simulink model "HybridFilter"  (R2022b)
settings: Solver=FixedStepDiscrete  StartTime=0.0  StopTime=10.0  RelTol=1e-3
libraries: simulink x1
settings Model: Creator=yuzehong  LastModifiedBy=yuzehong
settings OptimizationCC: DefaultParameterBehavior=Inlined  UseDivisionForNetSlopeComputation=on  GainParamInheritBuiltInType=on  UseFloatMulNetSlope=on  InlineInvariantSignals=on  PassReuseOutputArgsAs=Individual arguments  NoFixptDivByZeroProtection=on  EfficientFloat2IntCast=on  LifeSpan=1  OptimizeBlockOrder=speed  DifferentSizesBufferReuse=on  EfficientTunableParamExpr=on
settings DebuggingCC: ParameterTunabilityLossMsg=error
settings HardwareCC: ProdLongLongMode=on
settings SFSimCC: MATLABDynamicMemAlloc=off
settings RTWCC: Description=Embedded Coder  SystemTargetFile=ert.tlc  TemplateMakefile=ert_default_tmf
settings CodeAppCC: GenerateComments=off  IgnoreCustomStorageClasses=off  OperatorAnnotations=on  SimulinkDataObjDesc=on  SFDataObjDesc=on  CustomSymbolStrGlobalVar=rt$N$M  CustomSymbolStrType=$N$M  CustomSymbolStrFcn=$N$M$F  CustomSymbolStrMacro=$N$M  SimulinkBlockComments=off
settings ERTTargetCC: TargetLangStandard=C99 (ISO)  GenerateSampleERTMain=on  IncludeMdlTerminateFcn=off  CombineSignalStateStructs=on  SupportAbsoluteTime=off  CodeInterfacePackaging=Reusable function  SupportComplex=off  SupportNonInlinedSFcns=on  InlinedParameterPlacement=NonHierarchical  ERTCustomFileTemplate=example_file_process.tlc  ERTFilePackagingFormat=CompactWithDataFile

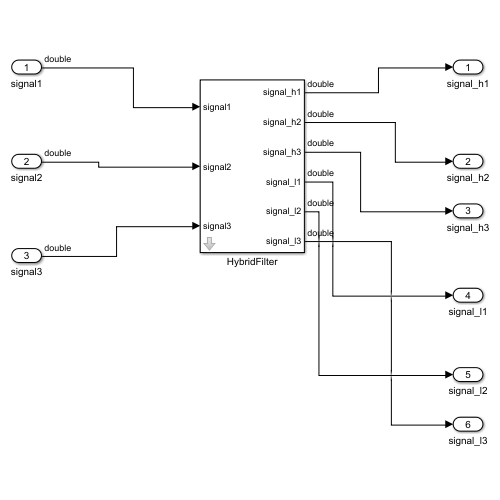
[thumbnail: Simulink's stored preview of the top-level diagram]
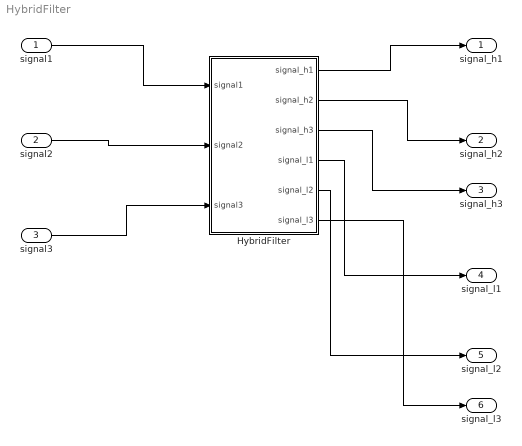
== system HybridFilter ==
  signal1 : Inport  OutDataTypeStr=double  PortDimensions=32
  signal2 : Inport  Port=2  OutDataTypeStr=double  PortDimensions=32
  signal3 : Inport  Port=3  OutDataTypeStr=double  PortDimensions=32
  HybridFilter : Subsystem  mask{length=32}
      mask DialogControl ParameterGroupVar Prompt: 参数
  signal_h1 : Outport
  signal_h2 : Outport  Port=2
  signal_h3 : Outport  Port=3
  signal_l1 : Outport  Port=4
  signal_l2 : Outport  Port=5
  signal_l3 : Outport  Port=6
  wires:
  signal1/1 -> HybridFilter/1(signal1)
  signal2/1 -> HybridFilter/2(signal2)
  signal3/1 -> HybridFilter/3(signal3)
  HybridFilter/1(signal_h1) -> signal_h1/1
  HybridFilter/2(signal_h2) -> signal_h2/1
  HybridFilter/3(signal_h3) -> signal_h3/1
  HybridFilter/4(signal_l1) -> signal_l1/1
  HybridFilter/5(signal_l2) -> signal_l2/1
  HybridFilter/6(signal_l3) -> signal_l3/1

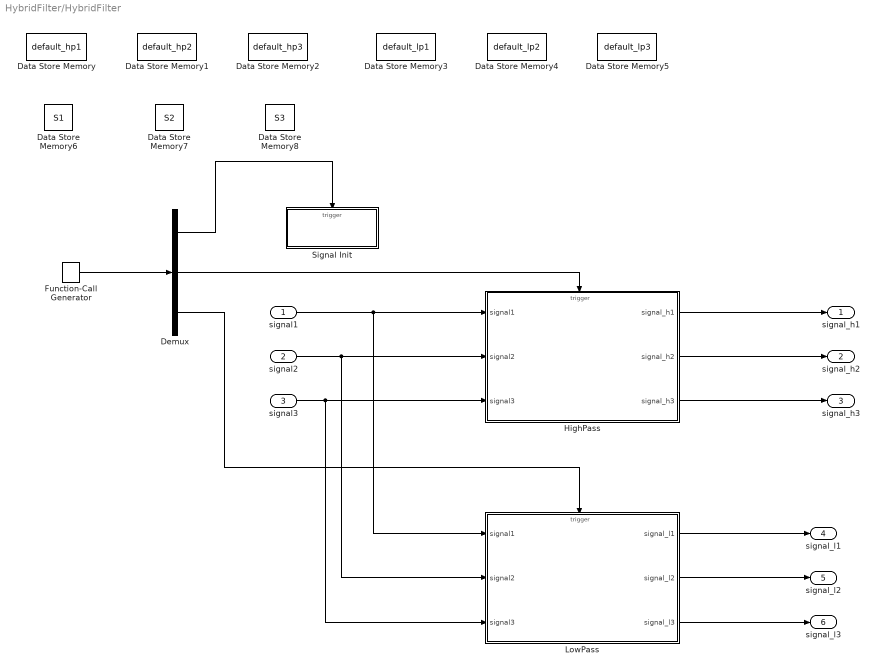
== system HybridFilter/HybridFilter ==
  signal1 : Inport  PortDimensions=length
  signal2 : Inport  Port=2  PortDimensions=length
  signal3 : Inport  Port=3  PortDimensions=length
  Data Store Memory : DataStoreMemory  DataStoreName=default_hp1  WriteAfterWriteMsg=warning  ShowAdditionalParam=off
  Data Store Memory1 : DataStoreMemory  DataStoreName=default_hp2  WriteAfterWriteMsg=warning  ShowAdditionalParam=off
  Data Store Memory2 : DataStoreMemory  DataStoreName=default_hp3  WriteAfterWriteMsg=warning  ShowAdditionalParam=off
  Data Store Memory3 : DataStoreMemory  DataStoreName=default_lp1  WriteAfterWriteMsg=warning  ShowAdditionalParam=off
  Data Store Memory4 : DataStoreMemory  DataStoreName=default_lp2  WriteAfterWriteMsg=warning  ShowAdditionalParam=off
  Data Store Memory5 : DataStoreMemory  DataStoreName=default_lp3  WriteAfterWriteMsg=warning  ShowAdditionalParam=off
  Data Store Memory6 : DataStoreMemory  DataStoreName=S1  WriteAfterWriteMsg=warning  ShowAdditionalParam=off  OutDataTypeStr=double  Dimensions=length
  Data Store Memory7 : DataStoreMemory  DataStoreName=S2  WriteAfterWriteMsg=warning  ShowAdditionalParam=off  OutDataTypeStr=double  Dimensions=length
  Data Store Memory8 : DataStoreMemory  DataStoreName=S3  WriteAfterWriteMsg=warning  ShowAdditionalParam=off  OutDataTypeStr=double  Dimensions=length
  Demux : Demux  Outputs=3
  Function-Call Generator : simulink/Ports & Subsystems/Function-Call Generator  sample_time=1  numberOfIterations=1  DisallowWideOutput=off
  HighPass : Subsystem
  LowPass : Subsystem
  Signal Init : Subsystem  TreatAsAtomicUnit=on
  signal_h1 : Outport
  signal_h2 : Outport  Port=2
  signal_h3 : Outport  Port=3
  signal_l1 : Outport  Port=4
  signal_l2 : Outport  Port=5
  signal_l3 : Outport  Port=6
  wires:
  Function-Call Generator/1 -> Demux/1
  Demux/1 -> Signal Init/Trigger
  signal1/1 -> LowPass/1(signal1), HighPass/1(signal1)
  signal2/1 -> LowPass/2(signal2), HighPass/2(signal2)
  signal3/1 -> LowPass/3(signal3), HighPass/3(signal3)
  HighPass/1(signal_h1) -> signal_h1/1
  HighPass/2(signal_h2) -> signal_h2/1
  HighPass/3(signal_h3) -> signal_h3/1
  Demux/2 -> HighPass/Trigger
  Demux/3 -> LowPass/Trigger
  LowPass/1(signal_l1) -> signal_l1/1
  LowPass/2(signal_l2) -> signal_l2/1
  LowPass/3(signal_l3) -> signal_l3/1

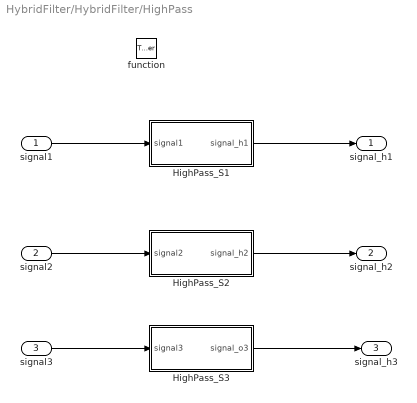
== system HybridFilter/HybridFilter/HighPass ==
  signal1 : Inport
  signal2 : Inport  Port=2
  signal3 : Inport  Port=3
  function : TriggerPort  TriggerType=function-call  VariantControl=(inherit)
  HighPass_S1 : Subsystem  TreatAsAtomicUnit=on
  HighPass_S2 : Subsystem  TreatAsAtomicUnit=on
  HighPass_S3 : Subsystem  TreatAsAtomicUnit=on
  signal_h1 : Outport
  signal_h2 : Outport  Port=2
  signal_h3 : Outport  Port=3
  wires:
  HighPass_S1/1(signal_h1) -> signal_h1/1
  HighPass_S2/1(signal_h2) -> signal_h2/1
  HighPass_S3/1(signal_o3) -> signal_h3/1
  signal1/1 -> HighPass_S1/1(signal1)
  signal2/1 -> HighPass_S2/1(signal2)
  signal3/1 -> HighPass_S3/1(signal3)

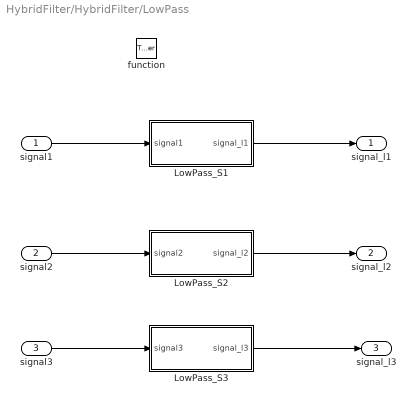
== system HybridFilter/HybridFilter/LowPass ==
  signal1 : Inport
  signal2 : Inport  Port=2
  signal3 : Inport  Port=3
  function : TriggerPort  TriggerType=function-call  VariantControl=(inherit)
  LowPass_S1 : Subsystem  TreatAsAtomicUnit=on
  LowPass_S2 : Subsystem  TreatAsAtomicUnit=on
  LowPass_S3 : Subsystem  TreatAsAtomicUnit=on
  signal_l1 : Outport
  signal_l2 : Outport  Port=2
  signal_l3 : Outport  Port=3
  wires:
  LowPass_S1/1(signal_l1) -> signal_l1/1
  LowPass_S2/1(signal_l2) -> signal_l2/1
  LowPass_S3/1(signal_l3) -> signal_l3/1
  signal1/1 -> LowPass_S1/1(signal1)
  signal2/1 -> LowPass_S2/1(signal2)
  signal3/1 -> LowPass_S3/1(signal3)

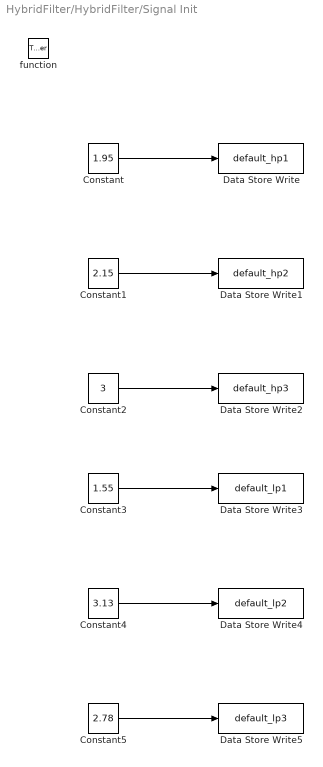
== system HybridFilter/HybridFilter/Signal Init ==
  function : TriggerPort  TriggerType=function-call  VariantControl=(inherit)
  Constant : Constant  Value=1.95  OutDataTypeStr=single
  Constant1 : Constant  Value=2.15  OutDataTypeStr=single
  Constant2 : Constant  Value=3  OutDataTypeStr=single
  Constant3 : Constant  Value=1.55  OutDataTypeStr=single
  Constant4 : Constant  Value=3.13  OutDataTypeStr=single
  Constant5 : Constant  Value=2.78  OutDataTypeStr=single
  Data Store Write : DataStoreWrite  DataStoreName=default_hp1  IndexOptions=Index vector (dialog)  Indices=1  OutputSizes=1
  Data Store Write1 : DataStoreWrite  DataStoreName=default_hp2  IndexOptions=Index vector (dialog)  Indices=1  OutputSizes=1
  Data Store Write2 : DataStoreWrite  DataStoreName=default_hp3  IndexOptions=Index vector (dialog)  Indices=1  OutputSizes=1
  Data Store Write3 : DataStoreWrite  DataStoreName=default_lp1  IndexOptions=Index vector (dialog)  Indices=1  OutputSizes=1
  Data Store Write4 : DataStoreWrite  DataStoreName=default_lp2  IndexOptions=Index vector (dialog)  Indices=1  OutputSizes=1
  Data Store Write5 : DataStoreWrite  DataStoreName=default_lp3  IndexOptions=Index vector (dialog)  Indices=1  OutputSizes=1
  wires:
  Constant/1 -> Data Store Write/1
  Constant1/1 -> Data Store Write1/1
  Constant2/1 -> Data Store Write2/1
  Constant5/1 -> Data Store Write5/1
  Constant4/1 -> Data Store Write4/1
  Constant3/1 -> Data Store Write3/1

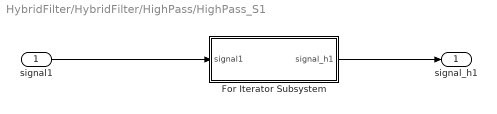
== system HybridFilter/HybridFilter/HighPass/HighPass_S1 ==
  signal1 : Inport
  For Iterator Subsystem : Subsystem  TreatAsAtomicUnit=on
  signal_h1 : Outport
  wires:
  signal1/1 -> For Iterator Subsystem/1(signal1)
  For Iterator Subsystem/1(signal_h1) -> signal_h1/1

== system HybridFilter/HybridFilter/HighPass/HighPass_S2 ==
  signal2 : Inport
  For Iterator Subsystem : Subsystem  TreatAsAtomicUnit=on
  signal_h2 : Outport
  wires:
  signal2/1 -> For Iterator Subsystem/1(signal2)
  For Iterator Subsystem/1(signal_h2) -> signal_h2/1

== system HybridFilter/HybridFilter/HighPass/HighPass_S3 ==
  signal3 : Inport
  For Iterator Subsystem : Subsystem  TreatAsAtomicUnit=on
  signal_o3 : Outport
  wires:
  For Iterator Subsystem/1(signal_o3) -> signal_o3/1
  signal3/1 -> For Iterator Subsystem/1(signal3)

== system HybridFilter/HybridFilter/LowPass/LowPass_S1 ==
  signal1 : Inport
  For Iterator Subsystem : Subsystem  TreatAsAtomicUnit=on
  signal_l1 : Outport
  wires:
  signal1/1 -> For Iterator Subsystem/1(signal1)
  For Iterator Subsystem/1(signal_l1) -> signal_l1/1

== system HybridFilter/HybridFilter/LowPass/LowPass_S2 ==
  signal2 : Inport
  For Iterator Subsystem : Subsystem  TreatAsAtomicUnit=on
  signal_l2 : Outport
  wires:
  signal2/1 -> For Iterator Subsystem/1(signal2)
  For Iterator Subsystem/1(signal_l2) -> signal_l2/1

== system HybridFilter/HybridFilter/LowPass/LowPass_S3 ==
  signal3 : Inport
  For Iterator Subsystem : Subsystem  TreatAsAtomicUnit=on
  signal_l3 : Outport
  wires:
  For Iterator Subsystem/1(signal_o3) -> signal_l3/1
  signal3/1 -> For Iterator Subsystem/1(signal3)

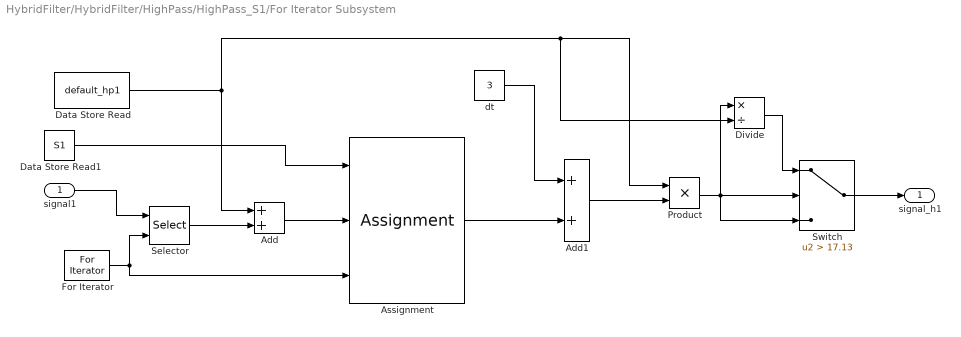
== system HybridFilter/HybridFilter/HighPass/HighPass_S1/For Iterator Subsystem ==
  signal1 : Inport
  Add : Sum
  Add1 : Sum
  Assignment : Assignment  IndexMode=Zero-based  DiagnosticForDimensions=Warning  IndexOptions=Index vector (port)  Indices=1  OutputSizes=1
  Data Store Read : DataStoreRead  DataStoreName=default_hp1  IndexOptions=Index vector (dialog)  Indices=1  OutputSizes=1
  Data Store Read1 : DataStoreRead  DataStoreName=S1  IndexOptions=Index vector (dialog)  Indices=1  OutputSizes=1
  Divide : Product  Inputs=*/
  For Iterator : ForIterator  IterationLimit=length  IndexMode=Zero-based
  Product : Product
  Selector : Selector  IndexMode=Zero-based  InputPortWidth=length  IndexOptions=Index vector (port)  Indices=[1 3]  OutputSizes=1
  Switch : Switch  Criteria=u2 > Threshold  Threshold=17.13  SaturateOnIntegerOverflow=off  InputSameDT=off
  dt : Constant  Value=3
  signal_h1 : Outport
  wires:
  For Iterator/1 -> Assignment/3, Selector/2
  Data Store Read1/1 -> Assignment/1
  Selector/1 -> Add/2
  Data Store Read/1 -> Divide/2, Product/1, Add/1
  Add/1 -> Assignment/2
  Assignment/1 -> Add1/2
  dt/1 -> Add1/1
  Add1/1 -> Product/2
  Product/1 -> Switch/2, Switch/3, Divide/1
  Switch/1 -> signal_h1/1
  Divide/1 -> Switch/1
  signal1/1 -> Selector/1

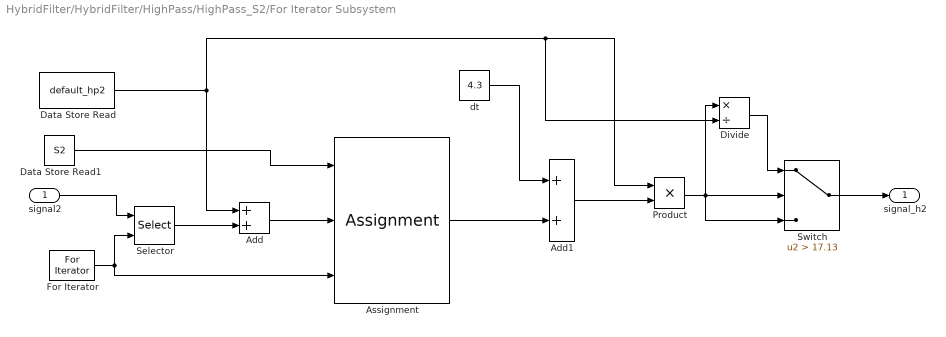
== system HybridFilter/HybridFilter/HighPass/HighPass_S2/For Iterator Subsystem ==
  signal2 : Inport
  Add : Sum
  Add1 : Sum
  Assignment : Assignment  IndexMode=Zero-based  DiagnosticForDimensions=Warning  IndexOptions=Index vector (port)  Indices=1  OutputSizes=1
  Data Store Read : DataStoreRead  DataStoreName=default_hp2  IndexOptions=Index vector (dialog)  Indices=1  OutputSizes=1
  Data Store Read1 : DataStoreRead  DataStoreName=S2  IndexOptions=Index vector (dialog)  Indices=1  OutputSizes=1
  Divide : Product  Inputs=*/
  For Iterator : ForIterator  IterationLimit=length  IndexMode=Zero-based
  Product : Product
  Selector : Selector  IndexMode=Zero-based  InputPortWidth=length  IndexOptions=Index vector (port)  Indices=[1 3]  OutputSizes=1
  Switch : Switch  Criteria=u2 > Threshold  Threshold=17.13  SaturateOnIntegerOverflow=off  InputSameDT=off
  dt : Constant  Value=4.3
  signal_h2 : Outport
  wires:
  For Iterator/1 -> Assignment/3, Selector/2
  signal2/1 -> Selector/1
  Selector/1 -> Add/2
  Data Store Read/1 -> Divide/2, Product/1, Add/1
  Add/1 -> Assignment/2
  Assignment/1 -> Add1/2
  dt/1 -> Add1/1
  Add1/1 -> Product/2
  Product/1 -> Switch/2, Switch/3, Divide/1
  Switch/1 -> signal_h2/1
  Divide/1 -> Switch/1
  Data Store Read1/1 -> Assignment/1

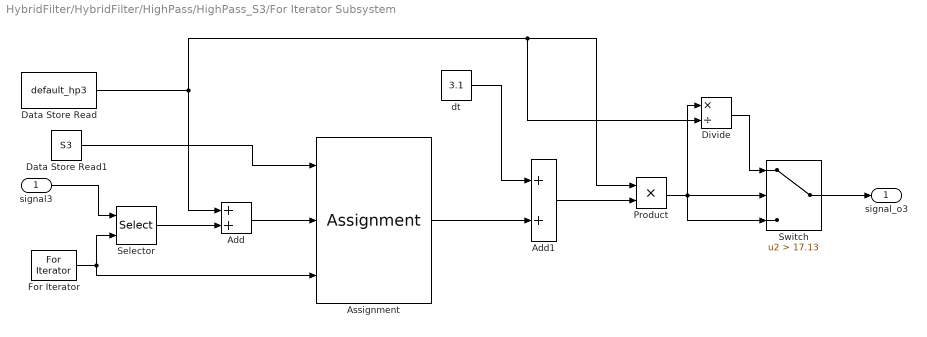
== system HybridFilter/HybridFilter/HighPass/HighPass_S3/For Iterator Subsystem ==
  signal3 : Inport
  Add : Sum
  Add1 : Sum
  Assignment : Assignment  IndexMode=Zero-based  DiagnosticForDimensions=Warning  IndexOptions=Index vector (port)  Indices=1  OutputSizes=1
  Data Store Read : DataStoreRead  DataStoreName=default_hp3  IndexOptions=Index vector (dialog)  Indices=1  OutputSizes=1
  Data Store Read1 : DataStoreRead  DataStoreName=S3  IndexOptions=Index vector (dialog)  Indices=1  OutputSizes=1
  Divide : Product  Inputs=*/
  For Iterator : ForIterator  IterationLimit=length  IndexMode=Zero-based
  Product : Product
  Selector : Selector  IndexMode=Zero-based  InputPortWidth=length  IndexOptions=Index vector (port)  Indices=[1 3]  OutputSizes=1
  Switch : Switch  Criteria=u2 > Threshold  Threshold=17.13  SaturateOnIntegerOverflow=off  InputSameDT=off
  dt : Constant  Value=3.1
  signal_o3 : Outport
  wires:
  For Iterator/1 -> Assignment/3, Selector/2
  signal3/1 -> Selector/1
  Selector/1 -> Add/2
  Data Store Read/1 -> Divide/2, Product/1, Add/1
  Add/1 -> Assignment/2
  Assignment/1 -> Add1/2
  dt/1 -> Add1/1
  Add1/1 -> Product/2
  Product/1 -> Switch/2, Switch/3, Divide/1
  Switch/1 -> signal_o3/1
  Divide/1 -> Switch/1
  Data Store Read1/1 -> Assignment/1

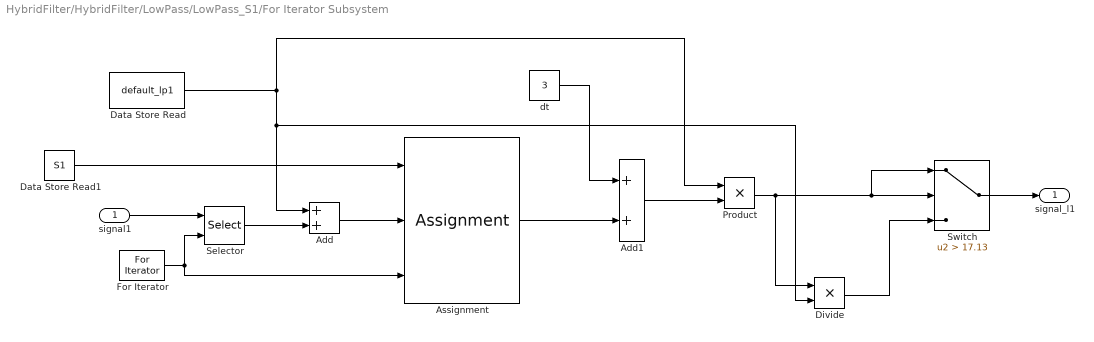
== system HybridFilter/HybridFilter/LowPass/LowPass_S1/For Iterator Subsystem ==
  signal1 : Inport
  Add : Sum
  Add1 : Sum
  Assignment : Assignment  IndexMode=Zero-based  DiagnosticForDimensions=Warning  IndexOptions=Index vector (port)  Indices=1  OutputSizes=1
  Data Store Read : DataStoreRead  DataStoreName=default_lp1  IndexOptions=Index vector (dialog)  Indices=1  OutputSizes=1
  Data Store Read1 : DataStoreRead  DataStoreName=S1  IndexOptions=Index vector (dialog)  Indices=1  OutputSizes=1
  Divide : Product  Inputs=**
  For Iterator : ForIterator  IterationLimit=length  IndexMode=Zero-based
  Product : Product
  Selector : Selector  IndexMode=Zero-based  InputPortWidth=length  IndexOptions=Index vector (port)  Indices=[1 3]  OutputSizes=1
  Switch : Switch  Criteria=u2 > Threshold  Threshold=17.13  SaturateOnIntegerOverflow=off  InputSameDT=off
  dt : Constant  Value=3
  signal_l1 : Outport
  wires:
  For Iterator/1 -> Assignment/3, Selector/2
  signal1/1 -> Selector/1
  Selector/1 -> Add/2
  Data Store Read/1 -> Divide/2, Add/1, Product/1
  Add/1 -> Assignment/2
  Assignment/1 -> Add1/2
  dt/1 -> Add1/1
  Add1/1 -> Product/2
  Product/1 -> Divide/1, Switch/1, Switch/2
  Switch/1 -> signal_l1/1
  Divide/1 -> Switch/3
  Data Store Read1/1 -> Assignment/1

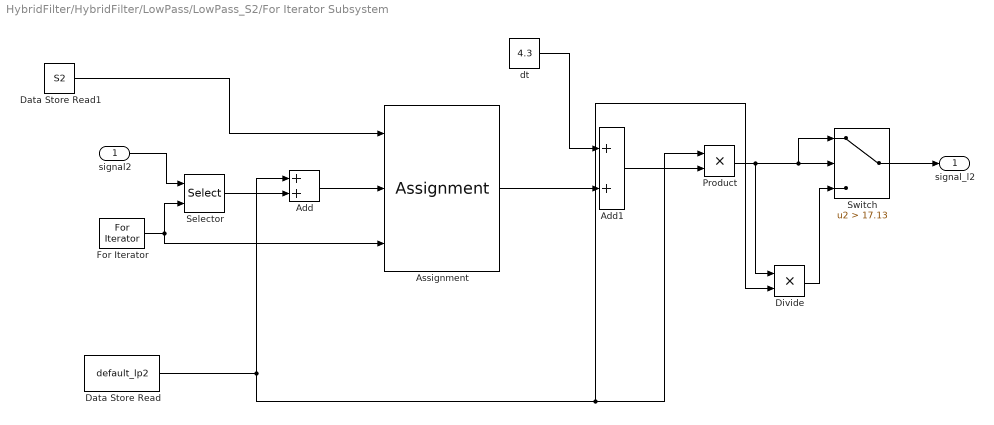
== system HybridFilter/HybridFilter/LowPass/LowPass_S2/For Iterator Subsystem ==
  signal2 : Inport
  Add : Sum
  Add1 : Sum
  Assignment : Assignment  IndexMode=Zero-based  DiagnosticForDimensions=Warning  IndexOptions=Index vector (port)  Indices=1  OutputSizes=1
  Data Store Read : DataStoreRead  DataStoreName=default_lp2  IndexOptions=Index vector (dialog)  Indices=1  OutputSizes=1
  Data Store Read1 : DataStoreRead  DataStoreName=S2  IndexOptions=Index vector (dialog)  Indices=1  OutputSizes=1
  Divide : Product  Inputs=**
  For Iterator : ForIterator  IterationLimit=length  IndexMode=Zero-based
  Product : Product
  Selector : Selector  IndexMode=Zero-based  InputPortWidth=length  IndexOptions=Index vector (port)  Indices=[1 3]  OutputSizes=1
  Switch : Switch  Criteria=u2 > Threshold  Threshold=17.13  SaturateOnIntegerOverflow=off  InputSameDT=off
  dt : Constant  Value=4.3
  signal_l2 : Outport
  wires:
  For Iterator/1 -> Assignment/3, Selector/2
  signal2/1 -> Selector/1
  Selector/1 -> Add/2
  Data Store Read/1 -> Add/1, Divide/2, Product/1
  Add/1 -> Assignment/2
  Assignment/1 -> Add1/2
  dt/1 -> Add1/1
  Add1/1 -> Product/2
  Product/1 -> Divide/1, Switch/1, Switch/2
  Switch/1 -> signal_l2/1
  Divide/1 -> Switch/3
  Data Store Read1/1 -> Assignment/1

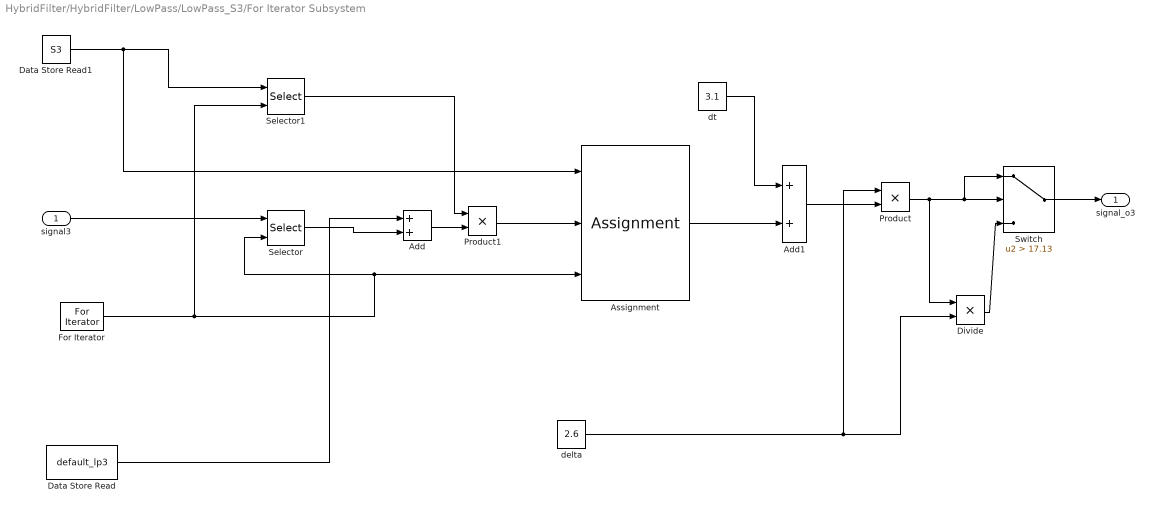
== system HybridFilter/HybridFilter/LowPass/LowPass_S3/For Iterator Subsystem ==
  signal3 : Inport
  Add : Sum
  Add1 : Sum
  Assignment : Assignment  IndexMode=Zero-based  DiagnosticForDimensions=Warning  IndexOptions=Index vector (port)  Indices=1  OutputSizes=1
  Data Store Read : DataStoreRead  DataStoreName=default_lp3  IndexOptions=Index vector (dialog)  Indices=1  OutputSizes=1
  Data Store Read1 : DataStoreRead  DataStoreName=S3  IndexOptions=Index vector (dialog)  Indices=1  OutputSizes=1
  Divide : Product  Inputs=**
  For Iterator : ForIterator  IterationLimit=length  IndexMode=Zero-based
  Product : Product
  Product1 : Product
  Selector : Selector  IndexMode=Zero-based  InputPortWidth=length  IndexOptions=Index vector (port)  Indices=[1 3]  OutputSizes=1
  Selector1 : Selector  IndexMode=Zero-based  InputPortWidth=length  IndexOptions=Index vector (port)  Indices=[1 3]  OutputSizes=1
  Switch : Switch  Criteria=u2 > Threshold  Threshold=17.13  SaturateOnIntegerOverflow=off  InputSameDT=off
  delta : Constant  Value=2.6
  dt : Constant  Value=3.1
  signal_o3 : Outport
  wires:
  For Iterator/1 -> Selector1/2, Selector/2, Assignment/3
  signal3/1 -> Selector/1
  Selector/1 -> Add/2
  Data Store Read/1 -> Add/1
  Assignment/1 -> Add1/2
  dt/1 -> Add1/1
  Add1/1 -> Product/2
  Product/1 -> Divide/1, Switch/1, Switch/2
  Switch/1 -> signal_o3/1
  Divide/1 -> Switch/3
  delta/1 -> Product/1, Divide/2
  Data Store Read1/1 -> Assignment/1, Selector1/1
  Add/1 -> Product1/2
  Selector1/1 -> Product1/1
  Product1/1 -> Assignment/2
